simulink model "SVPWM"  (R2018b)
settings: Solver=ode45  StartTime=0.0  StopTime=1  RelTol=1e-6
values from neighbouring files (symbols this model uses):
  fs = 10000    [Motor_parameters_project_modulation.m]
  J = 0.0151    [Motor_parameters_project_modulation.m]
  Lm = 0.38e-3    (= 0.00038)    [Motor_parameters_project_modulation.m]
  Lr = Lm + Ldr    (= 0.00041116)    [Motor_parameters_project_modulation.m]
  Ls = Lm + Lds    (= 0.00041116)    [Motor_parameters_project_modulation.m]
  Omegae = 2*pi*fn    (= 364.424747816)    [Motor_parameters_project_modulation.m]
  p = 2.0    (= 2)    [Motor_parameters_project_modulation.m]
  Rr = 2.69e-3    (= 0.00269)    [Motor_parameters_project_modulation.m]
  Rs = 2.5e-3    (= 0.0025)    [Motor_parameters_project_modulation.m]
  T_rated = Pn/(2*pi*nn/60)    (= 30.0363631473)    [Motor_parameters_project_modulation.m]
  Udc = 36    [Motor_parameters_project_modulation.m]
  Un = 24/sqrt(3)    [Motor_parameters_project_modulation.m]
undefined symbols (not defined in the file or in its folder): plecs
libraries: powerlib_meascontrol x1, simulink x1, powerlib x1
settings Model: SimulationMode=accelerator  Creator=estef  LastModifiedBy=estef
settings DebuggingCC: MaxConsecutiveZCsMsg=warning

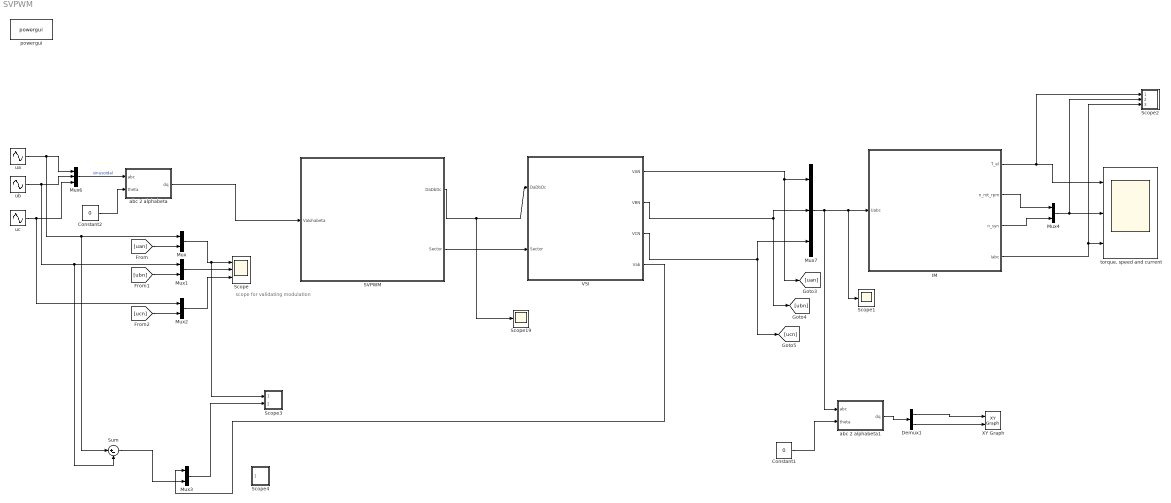
== system SVPWM ==
  note: scope for validating modulation
  Constant1 : Constant  Value=0
  Constant2 : Constant  Value=0
  Demux1 : Demux  Outputs=2
  "IM " : Subsystem
  Mux{,1..4} (5 alike) : Mux  Inputs=2
  Mux6 : Mux  Inputs=3
  Mux7 : Mux  Inputs=3
  "SVPWM " : Subsystem
  Scope : Scope  NumInputPorts=3
  Scope1 : Scope
  Scope19 : Scope
  Scope2 : Subsystem  LoadFcn=plecs('sl', 300);  InitFcn=plecs('sl', 314);  StartFcn=plecs('sl', 308);  StopFcn=plecs('sl', 309);  mask{Settings=}
      mask init:
      | plecs('sl', 315);
      settings: CopyFcn=plecs('sl', 303);  DeleteFcn=plecs('sl', 305);  UndoDeleteFcn=plecs('sl', 306);  PreSaveFcn=plecs('sl', 311);  NameChangeFcn=plecs('sl', 310);  DestroyFcn=plecs('sl', 307);  OpenFcn=plecs('sl', 302);  ErrorFcn=plerrorfcn
      mask Display: plot([0.1 0.9 0.9 0.1 0.1], [0.9 0.9 0.5 0.5 0.9])
  Scope3 : Subsystem  LoadFcn=plecs('sl', 300);  InitFcn=plecs('sl', 314);  StartFcn=plecs('sl', 308);  StopFcn=plecs('sl', 309);  mask{Settings=}
      mask init:
      | plecs('sl', 315);
      settings: CopyFcn=plecs('sl', 303);  DeleteFcn=plecs('sl', 305);  UndoDeleteFcn=plecs('sl', 306);  PreSaveFcn=plecs('sl', 311);  NameChangeFcn=plecs('sl', 310);  DestroyFcn=plecs('sl', 307);  OpenFcn=plecs('sl', 302);  ErrorFcn=plerrorfcn
      mask Display: plot([0.1 0.9 0.9 0.1 0.1], [0.9 0.9 0.5 0.5 0.9])
  Scope4 : Subsystem  LoadFcn=plecs('sl', 300);  InitFcn=plecs('sl', 314);  StartFcn=plecs('sl', 308);  StopFcn=plecs('sl', 309);  mask{Settings=}
      mask init:
      | plecs('sl', 315);
      settings: CopyFcn=plecs('sl', 303);  DeleteFcn=plecs('sl', 305);  UndoDeleteFcn=plecs('sl', 306);  PreSaveFcn=plecs('sl', 311);  NameChangeFcn=plecs('sl', 310);  DestroyFcn=plecs('sl', 307);  OpenFcn=plecs('sl', 302);  ErrorFcn=plerrorfcn
      mask Display: plot([0.1 0.9 0.9 0.1 0.1], [0.9 0.9 0.5 0.5 0.9])
  Sum : Sum  Inputs=|+-
  VSI : Subsystem
  XY Graph : simulink/Sinks/XY Graph  xmin=-1  xmax=1  ymin=-1  ymax=1  st=-1
  abc 2 alphabeta : Subsystem
  abc 2 alphabeta1 : Subsystem
  powergui : powerlib/powergui  Priority=1  SimulationMode=Continuous  SampleTime=50e-6  frequency=60  Iterations=50  frequencyindice=60  Pbase=100e6  ErrMax=1e-4  UnitsV=kV  UnitsW=MW  buscounter=0  FunctionMessages=off  echomessages=off  EnableUseOfTLC=off  CurrentSourceSwitches=off  DisableSnubberDevices=off  DisableRonSwitches=off  DisableVfSwitches=off  DisplayEquations=off  SolverType=Tustin/Backward Euler (TBE)  Interpol=off  ExternalGateDelay=off  methode=off  Ts=100  x0status=blocks  SPID=on  SwTol=0  HookPort=off  RestoreLinks=warning  ResistiveCurrentMeasurement=off  Frange=[0:2:500]  Ylog=off  Xlog=on  ShowGrid=off  save=off  variable=ZData  structure=phase_V  ZoomFFT=off  StartTime=0.1  cycles=10  DisplayStyle=1  fundamental=58  FreqAxis=off  MaxFrequency=1000  frequencyindicesteady=1  RmsSteady=1  display=off
  "torque, speed and current " : Scope  NumInputPorts=3
  ua : Sin  Amplitude=sqrt(2)*Un  Frequency=Omegae  SampleTime=0
  ub : Sin  Amplitude=sqrt(2)*Un  Frequency=Omegae  Phase=-2*pi/3  SampleTime=0
  uc : Sin  Amplitude=sqrt(2)*Un  Frequency=Omegae  Phase=2*pi/3  SampleTime=0
  wires:
  Mux7/1 -> abc 2 alphabeta1/1(abc), Scope1/1, "IM "/1("Uabc ")
  ub/1 -> Sum/2, Mux1/1, Mux6/2
  [ubn] -> Mux1/2
  [ucn] -> Mux2/2
  VSI/3(VCN) -> Mux7/3, [ucn]
  ua/1 -> Sum/1, Mux/1, Mux6/1
  [uan] -> Mux/2
  Mux1/1 -> Scope/2
  "IM "/1(T_el) -> Scope2/1(1), "torque, speed and current "/1
  uc/1 -> Mux2/1, Mux6/3
  VSI/1("VAN ") -> [uan], Mux7/1
  Mux2/1 -> Scope/3
  VSI/2("VBN ") -> Mux7/2, [ubn]
  Mux/1 -> Scope3/1(1), Scope/1
  "IM "/4(Iabc) -> Scope2/3(3), "torque, speed and current "/3
  Mux4/1 -> Scope2/2(2), "torque, speed and current "/2
  "IM "/2("n_rot_rpm ") -> Mux4/1
  "IM "/3("n_syn ") -> Mux4/2
  "SVPWM "/1(DaDbDc) -> Scope19/1, VSI/1(DaDbDc)
  VSI/4("Vab ") -> Mux3/1
  Constant2/1 -> abc 2 alphabeta/2(theta)
  Mux6/1 -> abc 2 alphabeta/1(abc)  "sinusoidal"
  abc 2 alphabeta/1(dq) -> "SVPWM "/1(Valohabeta)
  Constant1/1 -> abc 2 alphabeta1/2(theta)
  Demux1/2 -> XY Graph/2
  Demux1/1 -> XY Graph/1
  abc 2 alphabeta1/1(dq) -> Demux1/1
  Sum/1 -> Mux3/2
  Mux3/1 -> Scope3/2(2)
  "SVPWM "/2("Sector ") -> VSI/2("Sector ")

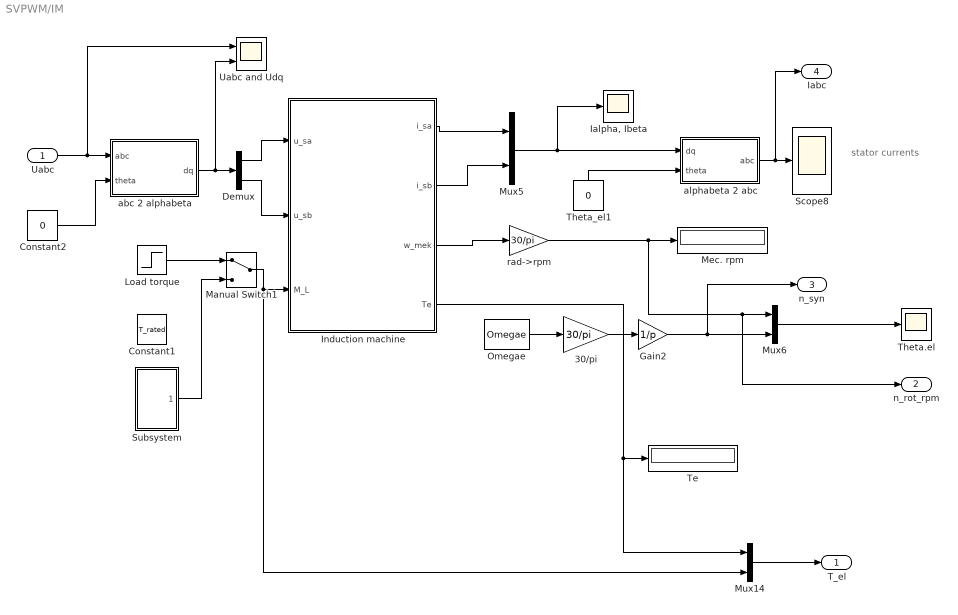
== system SVPWM/IM  ==
  note: stator currents
  "Uabc " : Inport
  30/pi : Gain  Gain=30/pi
  Constant1 : Constant  Value=T_rated
  Constant2 : Constant  Value=0
  Demux : Demux  Outputs=2
  Gain2 : Gain  Gain=1/p
  "Ialpha, Ibeta" : Scope
  "Induction machine " : Subsystem
  Load torque : Step  Time=0.3  After=T_rated  SampleTime=0
  Manual Switch1 : ManualSwitch
  Mec. rpm : Display
  Mux14 : Mux  Inputs=2
  Mux5 : Mux  Inputs=2
  Mux6 : Mux  Inputs=2
  Omegae : Constant  Value=Omegae
  Scope8 : Scope
  Subsystem : Subsystem
  Te : Display
  Theta.el : Scope
  Theta_el1 : Constant  Value=0
  Uabc and Udq : Scope  NumInputPorts=2
  abc 2 alphabeta : Subsystem
  alphabeta 2 abc : Subsystem
  rad->rpm : Gain  Gain=30/pi  SaturateOnIntegerOverflow=on  OutDataTypeStr=Inherit: Same as input  ParamDataTypeStr=Inherit: Same as input
  T_el : Outport
  "n_rot_rpm " : Outport  Port=2
  "n_syn " : Outport  Port=3
  Iabc : Outport  Port=4
  wires:
  rad->rpm/1 -> Mec. rpm/1, Mux6/1, "n_rot_rpm "/1
  "Induction machine "/4(Te) -> Mux14/1, Te/1
  Constant2/1 -> abc 2 alphabeta/2(theta)
  Manual Switch1/1 -> Mux14/2, "Induction machine "/3(M_L)
  Mux6/1 -> Theta.el/1
  abc 2 alphabeta/1(dq) -> Uabc and Udq/2, Demux/1
  Theta_el1/1 -> alphabeta 2 abc/2(theta)
  Mux14/1 -> T_el/1
  Mux5/1 -> "Ialpha, Ibeta"/1, alphabeta 2 abc/1(dq)
  "Induction machine "/1(i_sa) -> Mux5/1
  30/pi/1 -> Gain2/1
  "Induction machine "/3(w_mek) -> rad->rpm/1
  "Induction machine "/2(i_sb) -> Mux5/2
  Gain2/1 -> "n_syn "/1, Mux6/2
  Demux/1 -> "Induction machine "/1(u_sa)
  Omegae/1 -> 30/pi/1
  Demux/2 -> "Induction machine "/2(u_sb)
  "Uabc "/1 -> Uabc and Udq/1, abc 2 alphabeta/1(abc)
  alphabeta 2 abc/1(abc) -> Iabc/1, Scope8/1
  Subsystem/1(T_load) -> Manual Switch1/2
  Load torque/1 -> Manual Switch1/1

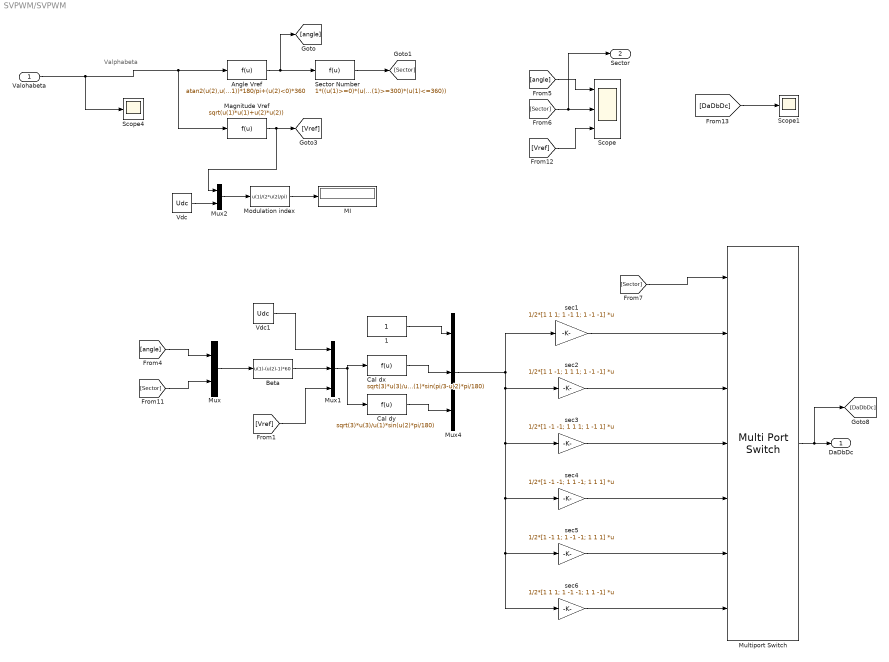
== system SVPWM/SVPWM  ==
  note: Valphabeta
  Valohabeta : Inport
  1 : Constant
  Angle Vref : Fcn  Expr=atan2(u(2),u(1))*180/pi+(u(2)<0)*360
  Beta : Fcn  Expr=u(1)-(u(2)-1)*60
  Cal dx : Fcn  Expr=sqrt(3)*u(3)/u(1)*sin(pi/3-u(2)*pi/180)
  Cal dy : Fcn  Expr=sqrt(3)*u(3)/u(1)*sin(u(2)*pi/180)
  MI : Display
  "Magnitude Vref " : Fcn  Expr=sqrt(u(1)*u(1)+u(2)*u(2))
  Modulation index : Fcn  Expr=u(1)/(2*u(2)/pi)
  Multiport Switch : MultiPortSwitch  Inputs=6
  Mux : Mux  Inputs=2
  Mux1 : Mux  Inputs=3
  Mux2 : Mux  Inputs=2
  Mux4 : Mux  Inputs=3
  Scope : Scope  NumInputPorts=3
  Scope1 : Scope
  Scope4 : Scope
  Sector Number : Fcn  Expr=1*((u(1)>=0)*(u(1)<60))+2*((u(1)>=60)*(u(1)<120))+3*((u(1)>=120)*(u(1)<180))+4*((u(1)>=180)*(u(1)<240))+5*((u(1)>=240)*(u(1)<300))+6*((u(1)>=300)*(u(1)<=360))
  Vdc : Constant  Value=Udc
  Vdc1 : Constant  Value=Udc
  sec1 : Gain  Gain=1/2*[1 1 1; 1 -1 1; 1 -1 -1]  Multiplication=Matrix(K*u)
  sec2 : Gain  Gain=1/2*[1 1 -1; 1 1 1; 1 -1 -1]  Multiplication=Matrix(K*u)
  sec3 : Gain  Gain=1/2*[1 -1 -1; 1 1 1; 1 -1 1]  Multiplication=Matrix(K*u)
  sec4 : Gain  Gain=1/2*[1 -1 -1; 1 1 -1; 1 1 1]  Multiplication=Matrix(K*u)
  sec5 : Gain  Gain=1/2*[1 -1 1; 1 -1 -1; 1 1 1]  Multiplication=Matrix(K*u)
  sec6 : Gain  Gain=1/2*[1 1 1; 1 -1 -1; 1 1 -1]  Multiplication=Matrix(K*u)
  DaDbDc : Outport
  "Sector " : Outport  Port=2
  wires:
  sec1/1 -> Multiport Switch/2
  Modulation index/1 -> MI/1
  sec3/1 -> Multiport Switch/4
  Mux2/1 -> Modulation index/1
  Sector Number/1 -> [Sector]
  sec4/1 -> Multiport Switch/5
  "Magnitude Vref "/1 -> Mux2/1, [Vref]
  Angle Vref/1 -> [angle], Sector Number/1
  sec5/1 -> Multiport Switch/6
  Vdc/1 -> Mux2/2
  sec2/1 -> Multiport Switch/3
  sec6/1 -> Multiport Switch/7
  [angle] -> Scope/1
  [Sector] -> "Sector "/1, Scope/2
  [Vref] -> Scope/3
  [DaDbDc] -> Scope1/1
  Mux/1 -> Beta/1
  [angle] -> Mux/1
  [Sector] -> Mux/2
  Beta/1 -> Mux1/2
  Vdc1/1 -> Mux1/1
  [Vref] -> Mux1/3
  Mux1/1 -> Cal dx/1, Cal dy/1
  1/1 -> Mux4/1
  Cal dx/1 -> Mux4/2
  Cal dy/1 -> Mux4/3
  Mux4/1 -> sec6/1, sec5/1, sec4/1, sec3/1, sec2/1, sec1/1
  Multiport Switch/1 -> DaDbDc/1, [DaDbDc]
  [Sector] -> Multiport Switch/1
  Valohabeta/1 -> Scope4/1, "Magnitude Vref "/1, Angle Vref/1

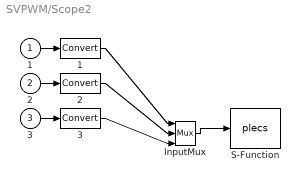
== system SVPWM/Scope2 ==
  1 : Inport
  2 : Inport  Port=2
  3 : Inport  Port=3
  " 1 " : DataTypeConversion  SaturateOnIntegerOverflow=on  RndMeth=Zero
  " 2 " : DataTypeConversion  SaturateOnIntegerOverflow=on  RndMeth=Zero
  " 3 " : DataTypeConversion  SaturateOnIntegerOverflow=on  RndMeth=Zero
  " InputMux " : Mux  Inputs=3
  " S-Function " : S-Function  FunctionName=plecs  SFunctionDeploymentMode=off  EnableBusSupport=off
  wires:
  " InputMux "/1 -> " S-Function "/1
  1/1 -> " 1 "/1
  " 1 "/1 -> " InputMux "/1
  2/1 -> " 2 "/1
  " 2 "/1 -> " InputMux "/2
  3/1 -> " 3 "/1
  " 3 "/1 -> " InputMux "/3

== system SVPWM/Scope3 ==
  1 : Inport
  2 : Inport  Port=2
  " 1 " : DataTypeConversion  SaturateOnIntegerOverflow=on  RndMeth=Zero
  " 2 " : DataTypeConversion  SaturateOnIntegerOverflow=on  RndMeth=Zero
  " InputMux " : Mux  Inputs=2
  " S-Function " : S-Function  FunctionName=plecs  SFunctionDeploymentMode=off  EnableBusSupport=off
  wires:
  " InputMux "/1 -> " S-Function "/1
  1/1 -> " 1 "/1
  " 1 "/1 -> " InputMux "/1
  2/1 -> " 2 "/1
  " 2 "/1 -> " InputMux "/2

== system SVPWM/Scope4 ==
  1 : Inport
  " InputMux " : Subsystem
      mask Display: disp('Mux')
  " S-Function " : S-Function  FunctionName=plecs  SFunctionDeploymentMode=off  EnableBusSupport=off
  wires:
  1/1 -> " InputMux "/1(In1)
  " InputMux "/1(Out) -> " S-Function "/1

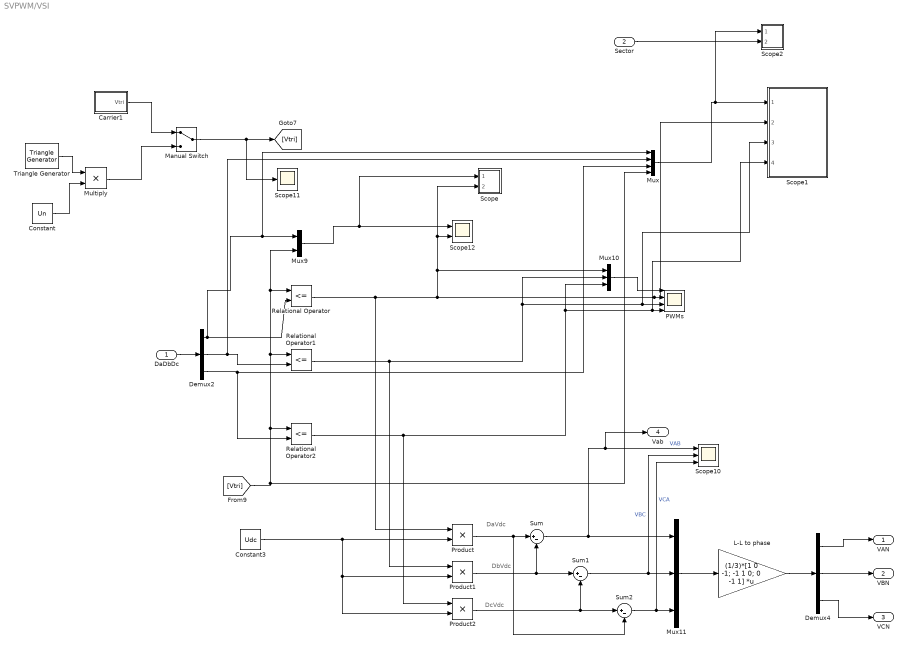
== system SVPWM/VSI ==
  note: DcVdc
  note: DaVdc
  note: DbVdc
  DaDbDc : Inport
  "Sector " : Inport  Port=2
  Carrier1 : Subsystem  mask{fsw=fs}
      mask prompts: fsw "switching frequency"
      mask init:
      | fsw2=fsw*2;
      | x=[0 1/4 3/4 1];
      | y=[0 -1     1    0];
      mask Display: plot([x  x+1 ],[y y])
  Constant : Constant  Value=Un
  Constant3 : Constant  Value=Udc
  Demux2 : Demux  Outputs=3
  Demux4 : Demux  Outputs=3
  "L-L to phase " : Gain  Gain=(1/3)*[1 0 -1; -1 1 0; 0 -1 1]  Multiplication=Matrix(K*u)
  Manual Switch : ManualSwitch
  Multiply : Product
  Mux : Mux
  Mux10 : Mux  Inputs=3
  Mux11 : Mux  Inputs=3
  Mux9 : Mux  Inputs=2
  "PWMs " : Scope  NumInputPorts=4
  Product : Product
  Product1 : Product
  Product2 : Product
  Relational Operator : RelationalOperator  Operator=<=  OutDataTypeStr=boolean  ZeroCross=off  RndMeth=Simplest
  Relational Operator1 : RelationalOperator  Operator=<=  OutDataTypeStr=boolean  ZeroCross=off  RndMeth=Simplest
  Relational Operator2 : RelationalOperator  Operator=<=  OutDataTypeStr=boolean  ZeroCross=off  RndMeth=Simplest
  Scope : Subsystem  LoadFcn=plecs('sl', 300);  InitFcn=plecs('sl', 314);  StartFcn=plecs('sl', 308);  StopFcn=plecs('sl', 309);  mask{Settings=}
      mask init:
      | plecs('sl', 315);
      settings: CopyFcn=plecs('sl', 303);  DeleteFcn=plecs('sl', 305);  UndoDeleteFcn=plecs('sl', 306);  PreSaveFcn=plecs('sl', 311);  NameChangeFcn=plecs('sl', 310);  DestroyFcn=plecs('sl', 307);  OpenFcn=plecs('sl', 302);  ErrorFcn=plerrorfcn
      mask Display: plot([0.1 0.9 0.9 0.1 0.1], [0.9 0.9 0.5 0.5 0.9])
  Scope1 : Subsystem  LoadFcn=plecs('sl', 300);  InitFcn=plecs('sl', 314);  StartFcn=plecs('sl', 308);  StopFcn=plecs('sl', 309);  mask{Settings=}
      mask init:
      | plecs('sl', 315);
      settings: CopyFcn=plecs('sl', 303);  DeleteFcn=plecs('sl', 305);  UndoDeleteFcn=plecs('sl', 306);  PreSaveFcn=plecs('sl', 311);  NameChangeFcn=plecs('sl', 310);  DestroyFcn=plecs('sl', 307);  OpenFcn=plecs('sl', 302);  ErrorFcn=plerrorfcn
      mask Display: plot([0.1 0.9 0.9 0.1 0.1], [0.9 0.9 0.5 0.5 0.9])
  Scope10 : Scope  NumInputPorts=3
  Scope11 : Scope
  Scope12 : Scope  NumInputPorts=2
  Scope2 : Subsystem  LoadFcn=plecs('sl', 300);  InitFcn=plecs('sl', 314);  StartFcn=plecs('sl', 308);  StopFcn=plecs('sl', 309);  mask{Settings=}
      mask init:
      | plecs('sl', 315);
      settings: CopyFcn=plecs('sl', 303);  DeleteFcn=plecs('sl', 305);  UndoDeleteFcn=plecs('sl', 306);  PreSaveFcn=plecs('sl', 311);  NameChangeFcn=plecs('sl', 310);  DestroyFcn=plecs('sl', 307);  OpenFcn=plecs('sl', 302);  ErrorFcn=plerrorfcn
      mask Display: plot([0.1 0.9 0.9 0.1 0.1], [0.9 0.9 0.5 0.5 0.9])
  Sum : Sum  Inputs=|+-
  Sum1 : Sum  Inputs=|+-
  Sum2 : Sum  Inputs=|+-
  Triangle Generator : powerlib_meascontrol/Pulse & Signal Generators/Triangle Generator  Freq=fs  Phase=0  Ts=0
  "VAN " : Outport
  "VBN " : Outport  Port=2
  VCN : Outport  Port=3
  "Vab " : Outport  Port=4
  wires:
  Sum1/1 -> Scope10/2, Mux11/2  "VBC"
  Constant3/1 -> Product2/2, Product1/2, Product/2
  Demux4/3 -> VCN/1
  Demux2/2 -> Mux/2, Relational Operator1/2
  Demux4/2 -> "VBN "/1
  Product/1 -> Sum/1, Sum2/2
  [Vtri] -> Mux/4, Relational Operator1/1, Mux9/2, Relational Operator/1, Relational Operator2/1
  DaDbDc/1 -> Demux2/1
  Demux2/1 -> Mux/1, Mux9/1, Relational Operator/2
  Demux4/1 -> "VAN "/1
  Relational Operator/1 -> Scope1/2(2), "PWMs "/2, Mux10/1, Scope/2(2), Scope12/2, Product/1
  Mux11/1 -> "L-L to phase "/1
  Product1/1 -> Sum1/1, Sum/2
  Product2/1 -> Sum2/1, Sum1/2
  Demux2/3 -> Mux/3, Relational Operator2/2
  Mux9/1 -> Scope/1(1), Scope12/1
  Relational Operator2/1 -> Product2/1, Scope1/4(4), "PWMs "/4, Mux10/3
  Sum/1 -> Mux11/1, "Vab "/1, Scope10/1  "VAB"
  Sum2/1 -> Scope10/3, Mux11/3  "VCA"
  "L-L to phase "/1 -> Demux4/1
  Relational Operator1/1 -> Scope1/3(3), "PWMs "/3, Mux10/2, Product1/1
  Carrier1/1(Vtri) -> Manual Switch/1
  Manual Switch/1 -> Scope11/1, [Vtri]
  Triangle Generator/1 -> Multiply/1
  Constant/1 -> Multiply/2
  Multiply/1 -> Manual Switch/2
  Mux10/1 -> "PWMs "/1
  Mux/1 -> Scope2/1(1), Scope1/1(1)
  "Sector "/1 -> Scope2/2(2)

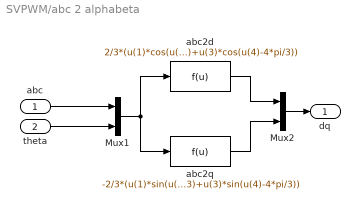
== system SVPWM/abc 2 alphabeta ==
  abc : Inport
  theta : Inport  Port=2
  Mux1 : Mux  Inputs=2
  Mux2 : Mux  Inputs=2
  abc2d : Fcn  Expr=2/3*(u(1)*cos(u(4))+u(2)*cos(u(4)-2*pi/3)+u(3)*cos(u(4)-4*pi/3))
  abc2q : Fcn  Expr=-2/3*(u(1)*sin(u(4))+u(2)*sin(u(4)-2*pi/3)+u(3)*sin(u(4)-4*pi/3))
  dq : Outport
  wires:
  abc/1 -> Mux1/1
  theta/1 -> Mux1/2
  Mux1/1 -> abc2d/1, abc2q/1
  abc2d/1 -> Mux2/1
  abc2q/1 -> Mux2/2
  Mux2/1 -> dq/1

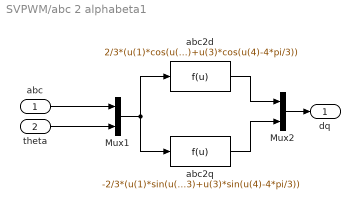
== system SVPWM/abc 2 alphabeta1 ==
  abc : Inport
  theta : Inport  Port=2
  Mux1 : Mux  Inputs=2
  Mux2 : Mux  Inputs=2
  abc2d : Fcn  Expr=2/3*(u(1)*cos(u(4))+u(2)*cos(u(4)-2*pi/3)+u(3)*cos(u(4)-4*pi/3))
  abc2q : Fcn  Expr=-2/3*(u(1)*sin(u(4))+u(2)*sin(u(4)-2*pi/3)+u(3)*sin(u(4)-4*pi/3))
  dq : Outport
  wires:
  abc/1 -> Mux1/1
  theta/1 -> Mux1/2
  Mux1/1 -> abc2d/1, abc2q/1
  abc2d/1 -> Mux2/1
  abc2q/1 -> Mux2/2
  Mux2/1 -> dq/1

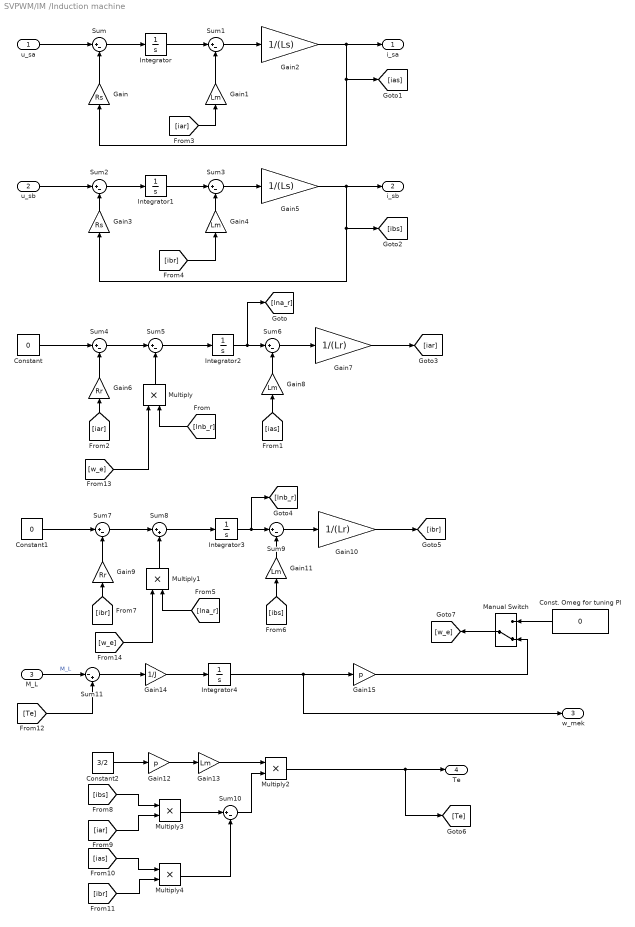
== system SVPWM/IM /Induction machine  ==
  u_sa : Inport
  u_sb : Inport  Port=2
  M_L : Inport  Port=3
  "Const. Omeg for tuning PI " : Constant  Value=0
  Constant : Constant  Value=0
  Constant1 : Constant  Value=0
  Constant2 : Constant  Value=3/2
  Gain : Gain  Gain=Rs
  Gain{1,4,8,11,13} (5 alike) : Gain  Gain=Lm
  Gain10 : Gain  Gain=1/(Lr)
  Gain12 : Gain  Gain=p
  Gain14 : Gain  Gain=1/J
  Gain15 : Gain  Gain=p
  Gain2 : Gain  Gain=1/(Ls)
  Gain3 : Gain  Gain=Rs
  Gain5 : Gain  Gain=1/(Ls)
  Gain6 : Gain  Gain=Rr
  Gain7 : Gain  Gain=1/(Lr)
  Gain9 : Gain  Gain=Rr
  Integrator{,1..4} (5 alike) : Integrator
  Manual Switch : ManualSwitch  CurrentSetting=0
  Multiply{,1..4} (5 alike) : Product
  Sum{,1..7,9..10} (10 alike) : Sum  Inputs=|+-
  Sum11 : Sum  Inputs=|-+
  Sum8 : Sum  Inputs=|++
  i_sa : Outport
  i_sb : Outport  Port=2
  w_mek : Outport  Port=3
  Te : Outport  Port=4
  wires:
  u_sa/1 -> Sum/1
  Gain/1 -> Sum/2
  Sum/1 -> Integrator/1
  Integrator/1 -> Sum1/1
  Gain1/1 -> Sum1/2
  Sum1/1 -> Gain2/1
  Gain2/1 -> [ias], Gain/1, i_sa/1
  Gain3/1 -> Sum2/2
  u_sb/1 -> Sum2/1
  Sum3/1 -> Gain5/1
  Gain4/1 -> Sum3/2
  Gain5/1 -> i_sb/1, [ibs], Gain3/1
  Sum2/1 -> Integrator1/1
  Integrator1/1 -> Sum3/1
  Constant/1 -> Sum4/1
  Gain6/1 -> Sum4/2
  Sum4/1 -> Sum5/1
  [lnb_r] -> Multiply/2
  Sum5/1 -> Integrator2/1
  Gain8/1 -> Sum6/2
  [ias] -> Gain8/1
  Integrator2/1 -> [lna_r], Sum6/1
  Sum6/1 -> Gain7/1
  Multiply/1 -> Sum5/2
  Gain7/1 -> [iar]
  [iar] -> Gain6/1
  [ibr] -> Gain4/1
  [iar] -> Gain1/1
  Gain11/1 -> Sum9/2
  Gain10/1 -> [ibr]
  [ibr] -> Gain9/1
  [ibs] -> Gain11/1
  Multiply1/1 -> Sum8/2
  Integrator3/1 -> [lnb_r], Sum9/1
  Sum7/1 -> Sum8/1
  [lna_r] -> Multiply1/2
  Gain9/1 -> Sum7/2
  Sum9/1 -> Gain10/1
  Sum8/1 -> Integrator3/1
  Constant1/1 -> Sum7/1
  Gain13/1 -> Multiply2/1
  Sum10/1 -> Multiply2/2
  [ibs] -> Multiply3/1
  [iar] -> Multiply3/2
  Multiply3/1 -> Sum10/1
  [ias] -> Multiply4/1
  [ibr] -> Multiply4/2
  Multiply4/1 -> Sum10/2
  Constant2/1 -> Gain12/1
  Gain12/1 -> Gain13/1
  Multiply2/1 -> [Te], Te/1
  [Te] -> Sum11/2
  M_L/1 -> Sum11/1  "M_L"
  Sum11/1 -> Gain14/1
  Gain14/1 -> Integrator4/1
  [w_e] -> Multiply/1
  [w_e] -> Multiply1/1
  "Const. Omeg for tuning PI "/1 -> Manual Switch/1
  Gain15/1 -> Manual Switch/2
  Manual Switch/1 -> [w_e]
  Integrator4/1 -> w_mek/1, Gain15/1

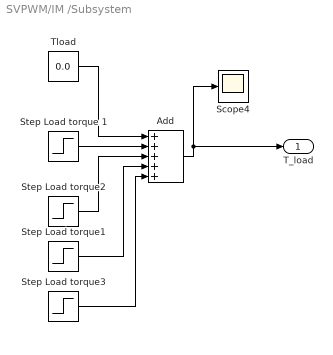
== system SVPWM/IM /Subsystem ==
  Add : Sum  Inputs=+++++
  Scope4 : Scope
  Step Load torque 1 : Step  Time=0.9  After=4  SampleTime=0
  Step Load torque1 : Step  Time=1.5  After=8  SampleTime=0
  Step Load torque2 : Step  Time=1.2  After=8  SampleTime=0
  Step Load torque3 : Step  Time=1.8  After=10  SampleTime=0
  Tload : Constant  Value=0.0
  T_load : Outport
  wires:
  Add/1 -> T_load/1, Scope4/1
  Step Load torque 1/1 -> Add/2
  Tload/1 -> Add/1
  Step Load torque2/1 -> Add/3
  Step Load torque1/1 -> Add/4
  Step Load torque3/1 -> Add/5

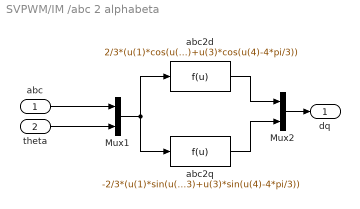
== system SVPWM/IM /abc 2 alphabeta ==
  abc : Inport
  theta : Inport  Port=2
  Mux1 : Mux  Inputs=2
  Mux2 : Mux  Inputs=2
  abc2d : Fcn  Expr=2/3*(u(1)*cos(u(4))+u(2)*cos(u(4)-2*pi/3)+u(3)*cos(u(4)-4*pi/3))
  abc2q : Fcn  Expr=-2/3*(u(1)*sin(u(4))+u(2)*sin(u(4)-2*pi/3)+u(3)*sin(u(4)-4*pi/3))
  dq : Outport
  wires:
  abc/1 -> Mux1/1
  theta/1 -> Mux1/2
  Mux1/1 -> abc2d/1, abc2q/1
  abc2d/1 -> Mux2/1
  abc2q/1 -> Mux2/2
  Mux2/1 -> dq/1

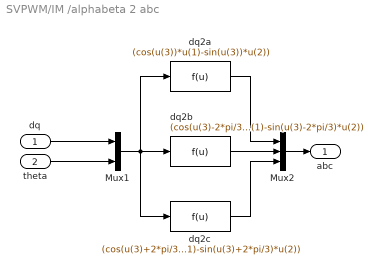
== system SVPWM/IM /alphabeta 2 abc ==
  dq : Inport
  theta : Inport  Port=2
  Mux1 : Mux  Inputs=2
  Mux2 : Mux  Inputs=3
  dq2a : Fcn  Expr=(cos(u(3))*u(1)-sin(u(3))*u(2))
  dq2b : Fcn  Expr=(cos(u(3)-2*pi/3)*u(1)-sin(u(3)-2*pi/3)*u(2))
  dq2c : Fcn  Expr=(cos(u(3)+2*pi/3)*u(1)-sin(u(3)+2*pi/3)*u(2))
  abc : Outport
  wires:
  Mux2/1 -> abc/1
  dq2b/1 -> Mux2/2
  dq2a/1 -> Mux2/1
  Mux1/1 -> dq2a/1, dq2c/1, dq2b/1
  theta/1 -> Mux1/2
  dq/1 -> Mux1/1
  dq2c/1 -> Mux2/3

== system SVPWM/Scope4/ InputMux  ==
  In1 : Inport
  Convert1 : DataTypeConversion  SaturateOnIntegerOverflow=on  RndMeth=Zero
  Mux : Mux  Inputs=1
  Out : Outport
  wires:
  Convert1/1 -> Mux/1
  In1/1 -> Convert1/1
  Mux/1 -> Out/1

== system SVPWM/VSI/Carrier1 ==
  note: set istart time 1/fsw/4
      | set initial IC 0.5
      | to have another waveform
      |  as shown on the block
  Constant : Constant
  Constant1 : Constant  Value=2*fs
  Integrator1 : Integrator
  Product : Product  SaturateOnIntegerOverflow=on  OutDataTypeStr=Inherit: Same as first input
  Pulse Generator : DiscretePulseGenerator  PulseType=Time based  Amplitude=2  Period=1/fsw  PulseWidth=50
  Sum : Sum  Inputs=|+-  SaturateOnIntegerOverflow=on
  Vtri : Outport  InitialOutput=0
  wires:
  Pulse Generator/1 -> Sum/1
  Constant/1 -> Sum/2
  Sum/1 -> Product/1
  Constant1/1 -> Product/2
  Product/1 -> Integrator1/1
  Integrator1/1 -> Vtri/1

== system SVPWM/VSI/Scope ==
  1 : Inport
  2 : Inport  Port=2
  " 1 " : DataTypeConversion  SaturateOnIntegerOverflow=on  RndMeth=Zero
  " 2 " : DataTypeConversion  SaturateOnIntegerOverflow=on  RndMeth=Zero
  " InputMux " : Mux  Inputs=2
  " S-Function " : S-Function  FunctionName=plecs  SFunctionDeploymentMode=off  EnableBusSupport=off
  wires:
  " InputMux "/1 -> " S-Function "/1
  1/1 -> " 1 "/1
  " 1 "/1 -> " InputMux "/1
  2/1 -> " 2 "/1
  " 2 "/1 -> " InputMux "/2

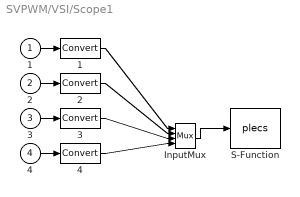
== system SVPWM/VSI/Scope1 ==
  1 : Inport
  2 : Inport  Port=2
  3 : Inport  Port=3
  4 : Inport  Port=4
  " 1 " : DataTypeConversion  SaturateOnIntegerOverflow=on  RndMeth=Zero
  " 2 " : DataTypeConversion  SaturateOnIntegerOverflow=on  RndMeth=Zero
  " 3 " : DataTypeConversion  SaturateOnIntegerOverflow=on  RndMeth=Zero
  " 4 " : DataTypeConversion  SaturateOnIntegerOverflow=on  RndMeth=Zero
  " InputMux " : Mux
  " S-Function " : S-Function  FunctionName=plecs  SFunctionDeploymentMode=off  EnableBusSupport=off
  wires:
  " InputMux "/1 -> " S-Function "/1
  1/1 -> " 1 "/1
  " 1 "/1 -> " InputMux "/1
  2/1 -> " 2 "/1
  " 2 "/1 -> " InputMux "/2
  3/1 -> " 3 "/1
  " 3 "/1 -> " InputMux "/3
  4/1 -> " 4 "/1
  " 4 "/1 -> " InputMux "/4

== system SVPWM/VSI/Scope2 ==
  1 : Inport
  2 : Inport  Port=2
  " 1 " : DataTypeConversion  SaturateOnIntegerOverflow=on  RndMeth=Zero
  " 2 " : DataTypeConversion  SaturateOnIntegerOverflow=on  RndMeth=Zero
  " InputMux " : Mux  Inputs=2
  " S-Function " : S-Function  FunctionName=plecs  SFunctionDeploymentMode=off  EnableBusSupport=off
  wires:
  " InputMux "/1 -> " S-Function "/1
  1/1 -> " 1 "/1
  " 1 "/1 -> " InputMux "/1
  2/1 -> " 2 "/1
  " 2 "/1 -> " InputMux "/2
